simulink library "mech_stewartplatform_leg"  (R2018a)
settings: Solver=VariableStepAuto  StartTime=0.0  StopTime=10.0  RelTol=1e-3
undefined symbols (not defined in the file): lower_leg_inertia, lower_leg_mass, upper_leg_inertia, upper_leg_mass
libraries: mblibv1 x7
Description:
  | Copyright 2008-2018 The MathWorks, Inc.
settings Model: ExtModeAutoUpdateStatusClock=off  Creator=MathWorks  LastModifiedBy=smiller
settings DataIOCC: SaveFormat=Array  SignalLoggingSaveFormat=ModelDataLogs
settings OptimizationCC: BlockReduction=off  BooleanDataType=off
settings DebuggingCC: SaveWithParameterizedLinksMsg=none  UnderspecifiedInitializationDetection=Classic  MergeDetectMultiDrivingBlocksExec=none  SignalResolutionControl=TryResolveAllWithWarning  MultiTaskCondExecSysMsg=none
settings HardwareCC: ProdBitPerPointer=32  ProdBitPerSizeT=32  ProdBitPerPtrDiffT=32  ProdLargestAtomicFloat=None  ProdIntDivRoundTo=Undefined  ProdEndianess=Unspecified  ProdWordSize=32  ProdHWDeviceType=32-bit Generic  TargetUnknown=on
settings ModelReferenceCC: PropagateSignalLabelsOutOfModel=off
settings CodeAppCC: StateflowObjectComments=on
settings ConfigComp: CovMetricSettings=dw  CovHtmlReporting=on  CovSaveCumulativeToWorkspaceVar=on  CovSaveSingleToWorkspaceVar=on  CovExternalEMLEnable=off

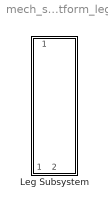
== system mech_stewartplatform_leg ==
  Leg Subsystem : Subsystem  mask{ln=1}
      mask prompts: ln "Leg Number"

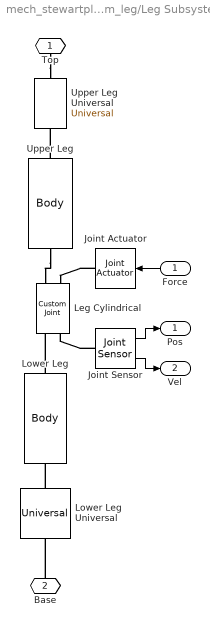
== system mech_stewartplatform_leg/Leg Subsystem ==
  Force : Inport  Description=Applies a force (N) to the prismatic axis
  Joint Actuator : mblibv1/Sensors &  Actuators/Joint Actuator  UpdateFromCAD=off  PhysicalDomain=Mechanical  PortType=blob  ActuationStyle=Force  AngleUnits=deg  ArcVelocityUnits=deg/s  ArcAccelerationUnits=deg/s^2  CoordPositionUnits=m  VelocityUnits=m/s  AccelerationUnits=m/s^2  ForceUnits=N  TorqueUnits=N-m  ActiveIO=off  Width=1  DialogClass=MechanicalActuatorBlock  Primitive=P1  ReferenceFrame=Absolute (INERTIAL)
      settings: SourceProductName=Simscape Multibody  SourceProductBaseCode=MS
  Joint Sensor : mblibv1/Sensors &  Actuators/Joint Sensor  UpdateFromCAD=off  PhysicalDomain=Mechanical  PortType=blob  Muxed=off  Pose=off  Angle=on  AngleUnits=deg  ArcVelocity=off  ArcVelocityUnits=deg/s  ArcAcceleration=off  ArcAccelerationUnits=deg/s^2  CoordPosition=on  CoordPositionUnits=m  Velocity=on  VelocityUnits=m/s  Acceleration=off  AccelerationUnits=m/s^2  Quaternion=on  QuaternionDT=off  QuaternionDDT=off  QuaternionUnits=off  OutputVector=[ 1 1 ]  ActiveIO=off  Width=1  DialogClass=MechanicalSensorBlock  Primitive=P1  Force=off  ForceUnits=N  Torque=off  TorqueUnits=N-m  ReferenceFrame=Absolute (INERTIAL)  ReactionSensedSide=Base  ReactionReferenceFrame=Absolute (World)  ReactionForce=off  ReactionForceUnits=N  ReactionMoment=off  ReactionMomentUnits=N-m
      settings: SourceProductName=Simscape Multibody  SourceProductBaseCode=MS
  Leg Cylindrical : mblibv1/Joints/Custom Joint  LConnTagsString=__newl0|SA1  RConnTagsString=__newr0|SA1  UpdateFromCAD=off  NumSAPorts=2  CutJoint=off  MarkAsCut=off  Primitives=revolute_prismatic  PrimitiveProps=R1$WORLD$cyl1(ln,:)$revolute#P1$WORLD$cyl1(ln,:)$prismatic  DialogClass=JointBlock  R1Axis=[0 0 1]  R2Axis=[]  R3Axis=[]  P1Axis=[]  P2Axis=[]  P3Axis=[]  SAxis=[]
      settings: SourceProductName=Simscape Multibody  SourceProductBaseCode=MS
  Lower Leg : mblibv1/Bodies/Body  LConnTagsString=CS1  RConnTagsString=CS3  UpdateFromCAD=off  DialogClass=MechanicalBodyBlock  Mass=lower_leg_mass  MassUnits=kg  InertiaUnits=kg*m^2  Inertia=lower_leg_inertia  Shape=Cylinder  ShapeDims=[1 1]  ShapeUnits=m  ShapeUse=false  Density=1  DensityUnits=kg/m^3  DensityUse=false  GraphicsMode=MACHINE_DEFAULT  BodyColorSelMode=MACHINE_DEFAULT  BodyColor=[1;0;0]  AttachedToCS=CG  CG=Left$CG$lower_leg(ln).origin$WORLD$WORLD$m$lower_leg(ln).rotation$3x3 Transform$deg$WORLD$false  WorkingFrames=Left$CS1$pos_base(ln,:)$WORLD$WORLD$m$lower_leg(ln).rotation$3x3 Transform$deg$WORLD$true#Right$CS3$(lower_leg(ln).end_point + upper_leg(ln).end_point)/2$WORLD$WORLD$m$lower_leg(ln).rotation$3x3 Transform$deg$WORLD$true#Right$CS2$lower_leg(ln).end_point$WORLD$WORLD$m$lower_leg(ln).rotation$3x3 Transform$deg$WORLD$false  CGPos=[0 0 0]  CGRot=[0 0 0]  CS0Pos=[]  CS0Rot=[]  CS1Pos=[0 0 0]  CS1Rot=[0 0 0]  CS2Pos=[0 0 0]  CS2Rot=[0 0 0]  CS3Pos=[]  CS3Rot=[]  CS4Pos=[]  CS4Rot=[]  CS5Pos=[]  CS5Rot=[]  CS6Pos=[]  CS6Rot=[]  CS7Pos=[]  CS7Rot=[]  CS8Pos=[]  CS8Rot=[]  CS9Pos=[]  CS9Rot=[]  CS10Pos=[]  CS10Rot=[]  CS11Pos=[]  CS11Rot=[]  CS12Pos=[]  CS12Rot=[]  CS13Pos=[]  CS13Rot=[]  CS14Pos=[]  CS14Rot=[]  CS15Pos=[]  CS15Rot=[]  CS16Pos=[]  CS16Rot=[]  CS17Pos=[]  CS17Rot=[]  CS18Pos=[]  CS18Rot=[]  CS19Pos=[]  CS19Rot=[]  CS20Pos=[]  CS20Rot=[]
      settings: SourceProductName=Simscape Multibody  SourceProductBaseCode=MS
  Lower Leg Universal : mblibv1/Joints/Universal  LConnTagsString=__newl0  RConnTagsString=__newr0  UpdateFromCAD=off  NumSAPorts=0  CutJoint=off  MarkAsCut=off  Primitives=revolute_revolute  PrimitiveProps=R1$WORLD$rev1(ln,:)$revolute#R2$WORLD$rev2(ln,:)$revolute  DialogClass=JointBlock  R1Axis=[0 0 1]  R2Axis=[0 1 0]
      settings: SourceProductName=Simscape Multibody  SourceProductBaseCode=MS
  Upper Leg : mblibv1/Bodies/Body  LConnTagsString=CS3  RConnTagsString=CS2  UpdateFromCAD=off  DialogClass=MechanicalBodyBlock  Mass=upper_leg_mass  MassUnits=kg  InertiaUnits=kg*m^2  Inertia=upper_leg_inertia  Shape=Cylinder  ShapeDims=[1 1]  ShapeUnits=m  ShapeUse=false  Density=1  DensityUnits=kg/m^3  DensityUse=false  GraphicsMode=MACHINE_DEFAULT  BodyColorSelMode=MACHINE_DEFAULT  BodyColor=[1;0;0]  AttachedToCS=CG  CG=Left$CG$upper_leg(ln).origin$WORLD$WORLD$m$upper_leg(ln).rotation$3x3 Transform$deg$WORLD$false  WorkingFrames=Left$CS3$(lower_leg(ln).end_point + upper_leg(ln).end_point)/2$WORLD$WORLD$m$upper_leg(ln).rotation$3x3 Transform$deg$WORLD$true#Left$CS1$upper_leg(ln).end_point$WORLD$WORLD$m$upper_leg(ln).rotation$3x3 Transform$deg$WORLD$false#Right$CS2$pos_top(ln,:)$WORLD$WORLD$m$upper_leg(ln).rotation$3x3 Transform$deg$WORLD$true  CGPos=[0 0 0]  CGRot=[0 0 0]  CS0Pos=[]  CS0Rot=[]  CS1Pos=[0 0 0]  CS1Rot=[0 0 0]  CS2Pos=[0 0 0]  CS2Rot=[0 0 0]  CS3Pos=[]  CS3Rot=[]  CS4Pos=[]  CS4Rot=[]  CS5Pos=[]  CS5Rot=[]  CS6Pos=[]  CS6Rot=[]  CS7Pos=[]  CS7Rot=[]  CS8Pos=[]  CS8Rot=[]  CS9Pos=[]  CS9Rot=[]  CS10Pos=[]  CS10Rot=[]  CS11Pos=[]  CS11Rot=[]  CS12Pos=[]  CS12Rot=[]  CS13Pos=[]  CS13Rot=[]  CS14Pos=[]  CS14Rot=[]  CS15Pos=[]  CS15Rot=[]  CS16Pos=[]  CS16Rot=[]  CS17Pos=[]  CS17Rot=[]  CS18Pos=[]  CS18Rot=[]  CS19Pos=[]  CS19Rot=[]  CS20Pos=[]  CS20Rot=[]
      settings: SourceProductName=Simscape Multibody  SourceProductBaseCode=MS
  Upper Leg Universal : mblibv1/Joints/Universal  LConnTagsString=__newl0  RConnTagsString=__newr0  UpdateFromCAD=off  NumSAPorts=0  CutJoint=off  MarkAsCut=off  Primitives=revolute_revolute  PrimitiveProps=R1$WORLD$rev3(ln,:)$revolute#R2$WORLD$rev4(ln,:)$revolute  DialogClass=JointBlock  R1Axis=[0 0 1]  R2Axis=[0 1 0]
      settings: SourceProductName=Simscape Multibody  SourceProductBaseCode=MS
  Top : PMIOPort  Side=Left
  Base : PMIOPort  Port=2  Side=Right
  Pos : Outport  Description=Senses position and velocity of the prismatic axis
  Vel : Outport  Description=Senses position and velocity of the prismatic axis  Port=2
  wires:
  Force/1 -> Joint Actuator/1
  Joint Sensor/1 -> Pos/1
  Joint Sensor/2 -> Vel/1
  connections:
  Lower Leg Universal/RConn1 -- Lower Leg/LConn1
  Upper Leg/RConn1 -- Upper Leg Universal/LConn1
  Top/RConn1 -- Upper Leg Universal/RConn1
  Base/RConn1 -- Lower Leg Universal/LConn1
  Joint Actuator/RConn1 -- Leg Cylindrical/RConn2
  Joint Sensor/LConn1 -- Leg Cylindrical/LConn2
  Lower Leg/RConn1 -- Leg Cylindrical/LConn1
  Upper Leg/LConn1 -- Leg Cylindrical/RConn1
